simulink model "Altitude_Hold"  (R2024a)
settings: Solver=VariableStepAuto  StartTime=0.0  StopTime=500  RelTol=1e-3
values from neighbouring files (symbols this model uses):
  CT = 0.20    (= 0.2)    [Estimation_AltHold.m]    (also in Estimation_AltHold_sim.m = 0.15)
  D = D*100    (= 8.89)    [Estimation_AltHold.m]    (also in Estimation_AltHold_sim.m)
  g = 9.81    [Estimation_AltHold.m]    (also in Estimation_AltHold_sim.m = 981)
  hoverOffset = 1275    [Estimation_AltHold.m]    (also in Estimation_AltHold_sim.m)
  KI_inner = KI*0.00012    (= 0.0018)    [Estimation_AltHold.m]    (also in Estimation_AltHold_sim.m)
  KI_outer = KI*0.0008    (= 0.012)    [Estimation_AltHold.m]    (also in Estimation_AltHold_sim.m)
  KP_inner = 15*0.005    (= 0.075)    [Estimation_AltHold.m]    (also in Estimation_AltHold_sim.m)
  KP_outer = 15*0.04    (= 0.6)    [Estimation_AltHold.m]    (also in Estimation_AltHold_sim.m)
  m = 0.300    (= 0.3)    [Estimation_AltHold.m]    (also in Estimation_AltHold_sim.m)
  PWM_max = 2000    [Estimation_AltHold.m]    (also in Estimation_AltHold_sim.m)
  PWM_min = 1000    [Estimation_AltHold.m]    (also in Estimation_AltHold_sim.m)
  rho = rho_m3 * 1e-6    (= 1.225e-06)    [Estimation_AltHold.m]    (also in Estimation_AltHold_sim.m)
  V_Bat = 16    [Estimation_AltHold.m]    (also in Estimation_AltHold_sim.m)
undefined symbols (not defined in the file or in its folder): DiscIntNeverNeededParam
libraries: cstblocks x2
settings Model: Creator=janick-dort  LastModifiedBy=janick-dort

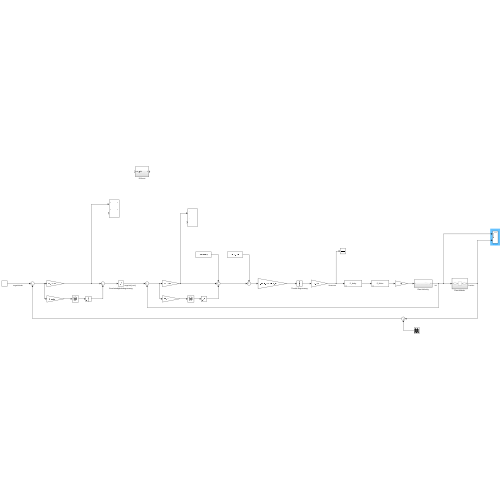
[thumbnail: Simulink's stored preview of the top-level diagram]
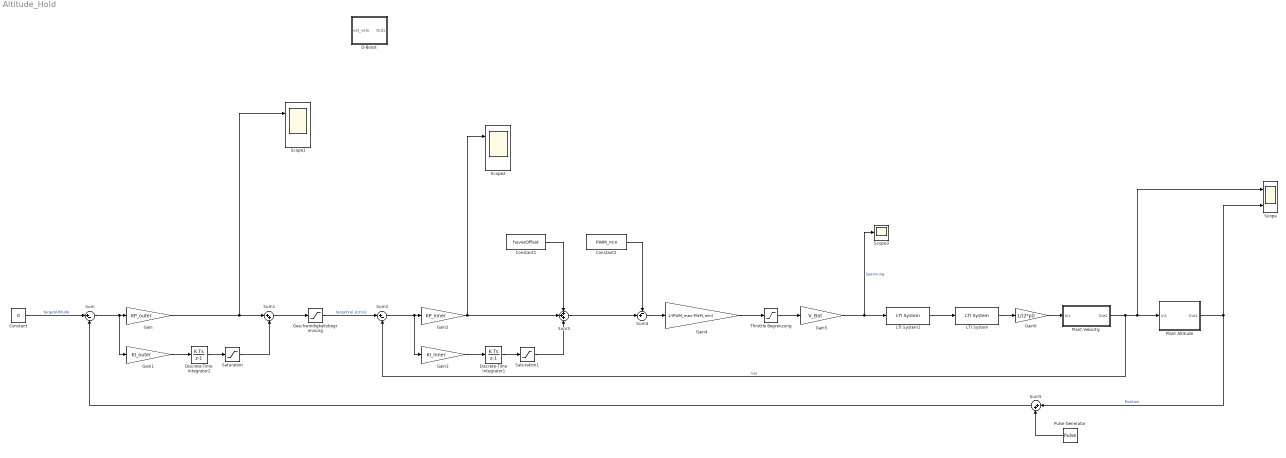
== system Altitude_Hold ==
  Constant : Constant  Value=0
  Constant1 : Constant  Value=hoverOffset
  Constant2 : Constant  Value=PWM_min
  D-Boost : Subsystem
  Discrete-Time Integrator1 : DiscreteIntegrator  SampleTime=0.01  ICPrevOutput=DiscIntNeverNeededParam  ICPrevScaledInput=DiscIntNeverNeededParam
  Discrete-Time Integrator2 : DiscreteIntegrator  SampleTime=0.01  ICPrevOutput=DiscIntNeverNeededParam  ICPrevScaledInput=DiscIntNeverNeededParam
  Gain : Gain  Gain=KP_outer
  Gain1 : Gain  Gain=KI_outer
  Gain2 : Gain  Gain=KP_inner
  Gain3 : Gain  Gain=KI_inner
  Gain4 : Gain  Gain=1/(PWM_max-PWM_min)
  Gain5 : Gain  Gain=V_Bat
  Gain6 : Gain  Gain=1/(2*pi)
  Geschwindigkeitsbegrenzung : Saturate  UpperLimit=1500  LowerLimit=-1500
  LTI System : cstblocks/LTI System  sys=P_Motor  IC=[]  PadeOrder=0
  LTI System1 : cstblocks/LTI System  sys=P_delay  IC=[]  PadeOrder=0
  Plant Altitude : Subsystem
  Plant Velocitiy : Subsystem
  Pulse Generator : DiscretePulseGenerator  PulseType=Time based  Amplitude=10  Period=0.01  PulseWidth=30
  Saturation : Saturate  UpperLimit=150  LowerLimit=-150
  Saturation1 : Saturate  UpperLimit=200  LowerLimit=-200
  Scope : Scope  NumInputPorts=2
  Scope1 : Scope  NumInputPorts=2
  Scope2 : Scope  NumInputPorts=2
  Scope3 : Scope
  Sum : Sum  Inputs=|+-
  Sum1 : Sum  Inputs=|++
  Sum2 : Sum  Inputs=|+-
  Sum3 : Sum  Inputs=+++
  Sum4 : Sum  Inputs=-+|
  Sum5 : Sum  Inputs=|++
  Throttle Begrenzung : Saturate  UpperLimit=1  LowerLimit=0
  wires:
  Constant/1 -> Sum/1  "targetAltitude"
  Sum/1 -> Gain1/1, Gain/1
  Gain1/1 -> Discrete-Time Integrator2/1
  Discrete-Time Integrator2/1 -> Saturation/1
  Gain/1 -> Sum1/1, Scope1/1
  Sum1/1 -> Geschwindigkeitsbegrenzung/1
  Sum2/1 -> Gain3/1, Gain2/1
  Gain3/1 -> Discrete-Time Integrator1/1
  Discrete-Time Integrator1/1 -> Saturation1/1
  Constant1/1 -> Sum3/1
  LTI System/1 -> Gain6/1
  Plant Velocitiy/1(Out1) -> Sum2/2, Plant Altitude/1(In1), Scope/1  "Vel"
  Plant Altitude/1(Out1) -> Sum5/1, Scope/2  "Position"
  Constant2/1 -> Sum4/1
  Sum4/1 -> Gain4/1
  Sum3/1 -> Sum4/2
  Gain4/1 -> Throttle Begrenzung/1
  Gain6/1 -> Plant Velocitiy/1(In1)
  Gain5/1 -> Scope3/1, LTI System1/1  "Spannung"
  LTI System1/1 -> LTI System/1
  Gain2/1 -> Scope2/1, Sum3/2
  Sum5/1 -> Sum/2
  Pulse Generator/1 -> Sum5/2
  Saturation1/1 -> Sum3/3
  Geschwindigkeitsbegrenzung/1 -> Sum2/1  "targetVel [cm/s]"
  Throttle Begrenzung/1 -> Gain5/1
  Saturation/1 -> Sum1/2

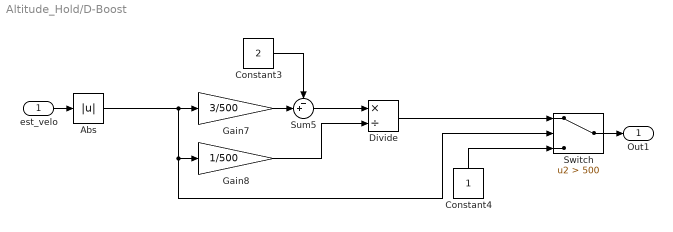
== system Altitude_Hold/D-Boost ==
  est_velo : Inport
  Abs : Abs  SaturateOnIntegerOverflow=off
  Constant3 : Constant  Value=2
  Constant4 : Constant
  Divide : Product  Inputs=*/
  Gain7 : Gain  Gain=3/500
  Gain8 : Gain  Gain=1/500
  Sum5 : Sum  Inputs=-+|
  Switch : Switch  Criteria=u2 > Threshold  Threshold=500  SaturateOnIntegerOverflow=off  InputSameDT=off
  Out1 : Outport
  wires:
  Constant4/1 -> Switch/3
  Abs/1 -> Switch/2, Gain8/1, Gain7/1
  Divide/1 -> Switch/1
  Sum5/1 -> Divide/1
  Gain7/1 -> Sum5/2
  Gain8/1 -> Divide/2
  Constant3/1 -> Sum5/1
  Switch/1 -> Out1/1
  est_velo/1 -> Abs/1

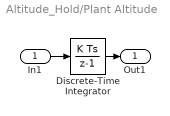
== system Altitude_Hold/Plant Altitude ==
  In1 : Inport
  Discrete-Time Integrator : DiscreteIntegrator  SampleTime=0.01  ICPrevOutput=DiscIntNeverNeededParam  ICPrevScaledInput=DiscIntNeverNeededParam
  Out1 : Outport
  wires:
  In1/1 -> Discrete-Time Integrator/1
  Discrete-Time Integrator/1 -> Out1/1

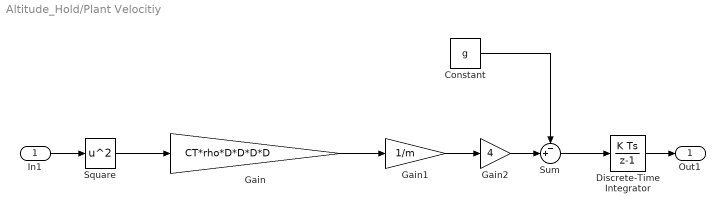
== system Altitude_Hold/Plant Velocitiy ==
  In1 : Inport
  Constant : Constant  Value=g
  Discrete-Time Integrator : DiscreteIntegrator  SampleTime=0.01  ICPrevOutput=DiscIntNeverNeededParam  ICPrevScaledInput=DiscIntNeverNeededParam
  Gain : Gain  Gain=CT*rho*D*D*D*D
  Gain1 : Gain  Gain=1/m
  Gain2 : Gain  Gain=4
  Square : Math  Operator=square
  Sum : Sum  Inputs=-+|
  Out1 : Outport
  wires:
  Gain/1 -> Gain1/1
  Gain1/1 -> Gain2/1
  Constant/1 -> Sum/1
  Sum/1 -> Discrete-Time Integrator/1
  Discrete-Time Integrator/1 -> Out1/1
  In1/1 -> Square/1
  Square/1 -> Gain/1
  Gain2/1 -> Sum/2
